simulink model "drone"  (Simulink 8.5)
settings: Solver=ode45  StartTime=0.0  StopTime=tsim  RelTol=1e-8  AbsTol=1e-12
undefined symbols (not defined in the file or in its folder): A, a_noise_seed, a_noise_var, a_scale, Cd, dx_init, enu2ecef, g, GPS_DT, GuideDt, h_noise_seed, h_noise_var, I, I_motor, IMU_DT, KaQ, KaR, KDhover, KIhover, Kir, KPhover, Kpr, Kpv, KQ, KR, KthQ, KthR, m, mag_bias, MAG_DT, mag_noise_seed, mag_noise_var, MaxPropRate, MaxPwmWidth, mean_a_bias, mean_w_bias, MinPwmWidth, mtow, P_init, Q, q0, qInit, R, r0, r1, r2, r3, r4, r_gps, RateToForce, Re, rho, Rmag, RunUpLimit, RunUpStartThrottle, tc, v0, v_noise_seed, v_noise_var, vc ... (+7)
libraries: simulink x13, SimLib x3
(part 2 of 2)

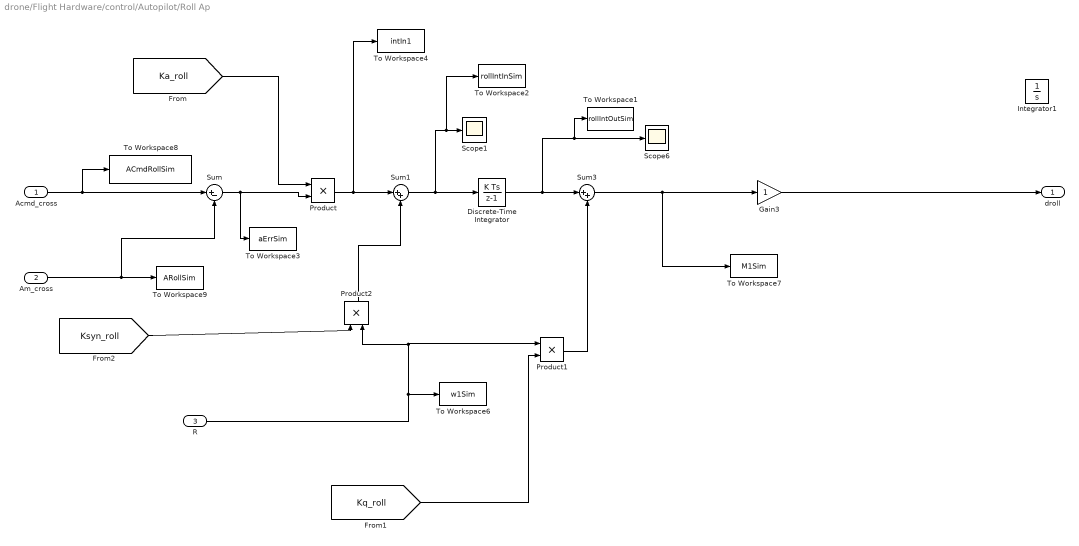
== system drone/Flight Hardware/control/Autopilot/Roll Ap ==
  Acmd_cross : Inport
  Am_cross : Inport  Port=2
  R : Inport  Port=3
  Discrete-Time Integrator : DiscreteIntegrator  InitialConditionSetting=State (most efficient)  SampleTime=IMU_DT
  Gain3 : Gain
  Integrator1 : Integrator
  Product : Product
  Product1 : Product
  Product2 : Product
  Scope1 : Scope
      settings: TimeRange=50  YMin=-10  YMax=8  SaveName=ScopeData15
  Scope6 : Scope
      settings: TimeRange=50  YMin=-0.005  YMax=0.03  SaveName=ScopeData115
  Sum : Sum  Inputs=|+-
  Sum1 : Sum  Inputs=|++
  Sum3 : Sum  Inputs=|++
  To Workspace1 : ToWorkspace  VariableName=rollIntOutSim  SampleTime=-1
  To Workspace2 : ToWorkspace  VariableName=rollIntInSim  SampleTime=-1
  To Workspace3 : ToWorkspace  VariableName=aErrSim  SampleTime=-1
  To Workspace4 : ToWorkspace  VariableName=intIn1  SampleTime=-1
  To Workspace6 : ToWorkspace  VariableName=w1Sim  SampleTime=-1
  To Workspace7 : ToWorkspace  VariableName=M1Sim  SampleTime=-1
  To Workspace8 : ToWorkspace  VariableName=ACmdRollSim  SampleTime=-1
  To Workspace9 : ToWorkspace  VariableName=ARollSim  SampleTime=-1
  droll : Outport
  wires:
  Am_cross/1 -> Sum/2, To Workspace9/1
  Product2/1 -> Sum1/2
  Sum1/1 -> Discrete-Time Integrator/1, To Workspace2/1, Scope1/1
  Product/1 -> To Workspace4/1, Sum1/1
  Discrete-Time Integrator/1 -> To Workspace1/1, Scope6/1, Sum3/1
  Product1/1 -> Sum3/2
  Sum3/1 -> To Workspace7/1, Gain3/1
  [Ka_roll] -> Product/1
  [Kq_roll] -> Product1/2
  R/1 -> To Workspace6/1, Product1/1, Product2/2
  [Ksyn_roll] -> Product2/1
  Acmd_cross/1 -> To Workspace8/1, Sum/1
  Gain3/1 -> droll/1
  Sum/1 -> To Workspace3/1, Product/2

== system drone/Flight Hardware/control/Autopilot/Throttle  ==
  ac : Inport
  am : Inport  Port=2
  Dot Product : DotProduct  InputSameDT=on  OutDataTypeStr=Inherit: Inherit via internal rule
  RunUp : Subsystem
  RunUp Logic : Subsystem
  Saturation : Saturate  UpperLimit=1  LowerLimit=0
  Scope{,1..3} (4 alike) : Scope
      Scope settings: TimeRange=10  YMin=0  YMax=0.2  SaveName=ScopeData2
      Scope1 settings: TimeRange=10  YMin=0.12445  YMax=0.13755  SaveName=ScopeData3
      Scope2 settings: TimeRange=10  YMin=9.7  YMax=11  SaveName=ScopeData68
      Scope3 settings: TimeRange=10  YMin=-106  YMax=-83  SaveName=ScopeData122
  Slope : Subsystem
  Sqrt : Sqrt  SaturateOnIntegerOverflow=on
  Step : Step  Time=15  Before=12  After=8  SampleTime=0.01
  Sum : Sum  Inputs=|++  AccumDataTypeStr=double  OutDataTypeStr=double
  To Workspace1 : ToWorkspace  VariableName=ThrottleSim  SampleTime=-1
  Throttle Cmd : Outport
  wires:
  Dot Product/1 -> Sqrt/1
  am/1 -> Dot Product/1, Dot Product/2
  RunUp Logic/2(runup x) -> Scope/1, RunUp/1(runUp)
  RunUp Logic/1(throttle x) -> Slope/3(runup)
  Sqrt/1 -> Scope2/1, RunUp Logic/1(am)
  RunUp/1(Out1) -> Scope1/1, Slope/2(RunUpValue), Sum/2
  Saturation/1 -> To Workspace1/1, Throttle Cmd/1
  Slope/1(Out1) -> Sum/1
  Sum/1 -> Scope3/1, Saturation/1
  ac/1 -> Slope/1(ac)

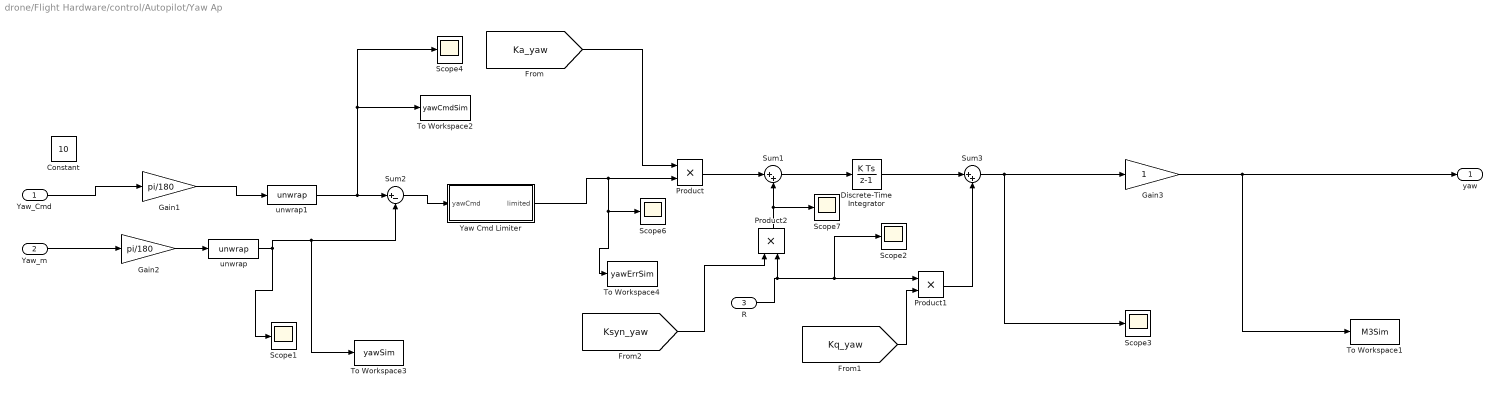
== system drone/Flight Hardware/control/Autopilot/Yaw Ap ==
  Yaw_Cmd : Inport
  Yaw_m : Inport  Port=2
  R : Inport  Port=3
  Constant : Constant  Value=10  SampleTime=IMU_DT
  Discrete-Time Integrator : DiscreteIntegrator  InitialConditionSetting=State (most efficient)  SampleTime=-1
  Gain1 : Gain  Gain=pi/180
  Gain2 : Gain  Gain=pi/180
  Gain3 : Gain
  Product : Product
  Product1 : Product
  Product2 : Product
  Scope{1..4,6..7} (6 alike) : Scope
      Scope1 settings: TimeRange=200  YMin=-0.05  YMax=0.4  SaveName=ScopeData15
      Scope2 settings: TimeRange=50  YMin=-2.5  YMax=37.5  SaveName=ScopeData48
      Scope3 settings: TimeRange=10  YMin=-7.034559643255292  YMax=12.94314381270903  SaveName=ScopeData12
      Scope4 settings: TimeRange=20  YMin=-0.006  YMax=0.006  SaveName=ScopeData119
      Scope6 settings: TimeRange=20  YMin=-0.006  YMax=0.006  SaveName=ScopeData52
      Scope7 settings: TimeRange=50  YMin=-2.5  YMax=37.5  SaveName=ScopeData53
  Sum1 : Sum  Inputs=|++
  Sum2 : Sum  Inputs=|+-
  Sum3 : Sum  Inputs=|++
  To Workspace1 : ToWorkspace  VariableName=M3Sim  SampleTime=-1
  To Workspace2 : ToWorkspace  VariableName=yawCmdSim  SampleTime=-1
  To Workspace3 : ToWorkspace  VariableName=yawSim  SampleTime=-1
  To Workspace4 : ToWorkspace  VariableName=yawErrSim  SampleTime=-1
  Yaw Cmd Limiter : Subsystem
  unwrap : SimLib/unwrap
  unwrap1 : SimLib/unwrap
  yaw : Outport
  wires:
  Product2/1 -> Scope7/1, Sum1/2
  Sum1/1 -> Discrete-Time Integrator/1
  Product/1 -> Sum1/1
  Discrete-Time Integrator/1 -> Sum3/1
  Product1/1 -> Sum3/2
  Sum3/1 -> Gain3/1, Scope3/1
  Gain3/1 -> To Workspace1/1, yaw/1
  [Ka_yaw] -> Product/1
  [Kq_yaw] -> Product1/2
  R/1 -> Product2/2, Scope2/1, Product1/1
  [Ksyn_yaw] -> Product2/1
  unwrap/1 -> To Workspace3/1, Sum2/2, Scope1/1
  unwrap1/1 -> Scope4/1, To Workspace2/1, Sum2/1
  Gain1/1 -> unwrap1/1
  Gain2/1 -> unwrap/1
  Yaw_m/1 -> Gain2/1
  Yaw_Cmd/1 -> Gain1/1
  Sum2/1 -> Yaw Cmd Limiter/1(yawCmd)
  Yaw Cmd Limiter/1("limited ") -> To Workspace4/1, Scope6/1, Product/2

== system drone/Flight Hardware/control/Guidance/v1 cmd ==
  r : Inport
  v : Inport  Port=2
  rc : Inport  Port=3
  vc : Inport  Port=4
  Embedded MATLAB Function2 : MATLAB Function  TreatAsAtomicUnit=on
  Gain : Gain  Gain=a_scale
  Mux1 : Mux  Inputs=2
  Scope{1..5,8} (6 alike) : Scope
      Scope1 settings: TimeRange=140  YMin=9.675  YMax=9.95  SaveName=ScopeData23
      Scope2 settings: TimeRange=2.391750639737455  YMin=-0.00131617173055854  YMax=0.0006389084610017104  SaveName=ScopeData117
      Scope3 settings: TimeRange=80  YMin=-0.5  YMax=10  SaveName=ScopeData31
      Scope4 settings: TimeRange=140  YMin=8  YMax=24  SaveName=ScopeData39
      Scope5 settings: TimeRange=140  YMin=-5e+09  YMax=1e+10  SaveName=ScopeData84
      Scope8 settings: TimeRange=140  YMin=8.75  YMax=9.5  SaveName=ScopeData114
  Subsystem : Subsystem
  Subsystem2 : Subsystem
  Subsystem3 : Subsystem
  Sum4 : Sum  Inputs=+++
  To Workspace1 : ToWorkspace  VariableName=vErr  SampleTime=-1
  To Workspace2 : ToWorkspace  VariableName=rErr  SampleTime=-1
  To Workspace3 : ToWorkspace  VariableName=aCurve  SampleTime=-1
  To Workspace4 : ToWorkspace  VariableName=hErr  SampleTime=-1
  To Workspace5 : ToWorkspace  VariableName=vH  SampleTime=-1
  To Workspace6 : ToWorkspace  VariableName=accelCmd  SampleTime=-1
  To Workspace7 : ToWorkspace  VariableName=hAccelCmd  SampleTime=-1
  acmd : Outport
  f tot : Outport  Port=2
  wires:
  Subsystem/1(ftot) -> Mux1/2, To Workspace7/1, Scope1/1
  Sum4/1 -> Mux1/1
  r/1 -> Subsystem3/1(r)
  rc/1 -> Subsystem3/2(rc)
  v/1 -> Subsystem3/4(v)
  vc/1 -> Subsystem3/3(vc)
  Subsystem3/4(herr) -> To Workspace4/1, Subsystem/1(herr), Scope5/1
  Subsystem3/3(acurve) -> To Workspace3/1, Sum4/3, Scope8/1
  Subsystem3/1(eR) -> To Workspace2/1, Subsystem2/1(eP)
  Embedded MATLAB Function2/1(ftot) -> f tot/1, Scope4/1
  Gain/1 -> Embedded MATLAB Function2/1(acmd), acmd/1
  Mux1/1 -> Gain/1, Scope3/1
  Subsystem3/2("ev ") -> To Workspace1/1, Subsystem2/2(v)
  Subsystem2/1(vc) -> To Workspace6/1, Sum4/1
  Subsystem3/5(vh) -> To Workspace5/1, Subsystem/2(vh)

== system drone/Flight Hardware/state estimator1/Subsystem/solve direction cosine matrix ==
  quat : Inport
  C11 : Fcn  Expr=1-(2*u[2]*u[2]) - (2*u[3]*u[3])
  C12 : Fcn  Expr=2*( u[1]*u[2] - u[3]*u[4])
  C13 : Fcn  Expr=2*( u[3]*u[1] + u[2]*u[4])
  C21 : Fcn  Expr=2*( u[1]*u[2] + u[3]*u[4])
  C22 : Fcn  Expr=1-(2*u[1]*u[1]) - (2*u[3]*u[3])
  C23 : Fcn  Expr=2*( u[3]*u[2] - u[1]*u[4])
  C31 : Fcn  Expr=2*( u[1]*u[3] - u[2]*u[4])
  C32 : Fcn  Expr=2*( u[3]*u[2] + u[1]*u[4])
  C33 : Fcn  Expr=1-(2*u[2]*u[2]) - (2*u[1]*u[1])
  Gain1 : Gain  Gain=180/pi
  Gain2 : Gain  Gain=-1
  Gain3 : Gain  Gain=-1
  MATLAB Function : MATLAB Function  TreatAsAtomicUnit=on
  Mux : Mux  Inputs=3
  nutation : Trigonometry  Operator=asin
  precession : Trigonometry  Operator=atan2
  spin : Trigonometry  Operator=atan2
  C : Outport
  roll pitch yaw : Outport  Port=2
  wires:
  quat/1 -> C13/1, C11/1, C12/1, C21/1, C22/1, C23/1, C31/1, C33/1, C32/1
  C11/1 -> MATLAB Function/1(C11)
  C12/1 -> MATLAB Function/2(C12), Gain2/1
  C13/1 -> MATLAB Function/3(C13)
  C21/1 -> MATLAB Function/4(C21)
  C22/1 -> MATLAB Function/5(C22), spin/2
  C23/1 -> MATLAB Function/6(C23)
  C31/1 -> MATLAB Function/7(C31), Gain3/1
  C32/1 -> MATLAB Function/8(C32), nutation/1
  C33/1 -> MATLAB Function/9(C33), precession/2
  Gain1/1 -> roll pitch yaw/1
  Mux/1 -> Gain1/1
  Gain2/1 -> spin/1
  Gain3/1 -> precession/1
  nutation/1 -> Mux/1
  spin/1 -> Mux/3
  precession/1 -> Mux/2
  MATLAB Function/1(R) -> C/1

== system drone/Physics Modeling/Equations of Motion/Subsystem/solve direction cosine matrix ==
  quat : Inport
  C11 : Fcn  Expr=1-(2*u[2]*u[2]) - (2*u[3]*u[3])
  C12 : Fcn  Expr=2*( u[1]*u[2] - u[3]*u[4])
  C13 : Fcn  Expr=2*( u[3]*u[1] + u[2]*u[4])
  C21 : Fcn  Expr=2*( u[1]*u[2] + u[3]*u[4])
  C22 : Fcn  Expr=1-(2*u[1]*u[1]) - (2*u[3]*u[3])
  C23 : Fcn  Expr=2*( u[3]*u[2] - u[1]*u[4])
  C31 : Fcn  Expr=2*( u[1]*u[3] - u[2]*u[4])
  C32 : Fcn  Expr=2*( u[3]*u[2] + u[1]*u[4])
  C33 : Fcn  Expr=1-(2*u[2]*u[2]) - (2*u[1]*u[1])
  Gain1 : Gain  Gain=360/(2*pi)
  Gain2 : Gain  Gain=-1
  Gain3 : Gain  Gain=-1
  MATLAB Function : MATLAB Function  TreatAsAtomicUnit=on
  Mux : Mux  Inputs=3
  nutation : Trigonometry  Operator=asin
  precession : Trigonometry  Operator=atan2
  spin : Trigonometry  Operator=atan2
  C : Outport
  roll pitch yaw : Outport  Port=2
  wires:
  quat/1 -> C13/1, C11/1, C12/1, C21/1, C22/1, C23/1, C31/1, C33/1, C32/1
  C11/1 -> MATLAB Function/1(C11)
  C12/1 -> MATLAB Function/2(C12), Gain2/1
  C13/1 -> MATLAB Function/3(C13)
  C21/1 -> MATLAB Function/4(C21)
  C22/1 -> MATLAB Function/5(C22), spin/2
  C23/1 -> MATLAB Function/6(C23)
  C31/1 -> MATLAB Function/7(C31), Gain3/1
  C32/1 -> MATLAB Function/8(C32), nutation/1
  C33/1 -> MATLAB Function/9(C33), precession/2
  Gain1/1 -> roll pitch yaw/1
  Mux/1 -> Gain1/1
  Gain2/1 -> spin/1
  Gain3/1 -> precession/1
  nutation/1 -> Mux/1
  spin/1 -> Mux/3
  precession/1 -> Mux/2
  MATLAB Function/1(R) -> C/1

== system drone/Physics Modeling/Props/Rate to Force/location moment ==
  F1 : Inport
  F2 : Inport  Port=2
  F3 : Inport  Port=3
  F4 : Inport  Port=4
  Constant : Constant  Value=r1
  Constant1 : Constant  Value=r2
  Constant2 : Constant  Value=r3
  Constant3 : Constant  Value=r4
  MATLAB Function : MATLAB Function  TreatAsAtomicUnit=on
  MATLAB Function1 : MATLAB Function  TreatAsAtomicUnit=on
  MATLAB Function2 : MATLAB Function  TreatAsAtomicUnit=on
  MATLAB Function3 : MATLAB Function  TreatAsAtomicUnit=on
  Scope{1..4} (4 alike) : Scope
      Scope1 settings: YMin=-1  YMax=1  SaveName=ScopeData17
      Scope2 settings: TimeRange=50  YMin=-1  YMax=1  SaveName=ScopeData16
      Scope3 settings: TimeRange=50  YMin=-1  YMax=1  SaveName=ScopeData18
      Scope4 settings: TimeRange=50  YMin=-1  YMax=1  SaveName=ScopeData19
  Sum : Sum  Inputs=++++
  M : Outport
  wires:
  F2/1 -> MATLAB Function1/2(u2)
  F1/1 -> MATLAB Function/2(u2)
  Constant/1 -> MATLAB Function/1(u1)
  Sum/1 -> M/1
  MATLAB Function/1(y) -> Scope2/1, Sum/1
  MATLAB Function1/1(y) -> Sum/2, Scope1/1
  MATLAB Function2/1(y) -> Scope3/1, Sum/3
  MATLAB Function3/1(y) -> Sum/4, Scope4/1
  Constant1/1 -> MATLAB Function1/1(u1)
  Constant2/1 -> MATLAB Function2/1(u1)
  F3/1 -> MATLAB Function2/2(u2)
  F4/1 -> MATLAB Function3/2(u2)
  Constant3/1 -> MATLAB Function3/1(u1)

== system drone/Physics Modeling/Props/Rate to Force/location moment1 ==
  F : Inport
  Constant : Constant  Value=0
  Mux : Mux  Inputs=3
  F1 : Outport
  wires:
  Constant/1 -> Mux/2, Mux/1
  F/1 -> Mux/3
  Mux/1 -> F1/1

== system drone/Physics Modeling/Props/Rate to Force/location moment2 ==
  F : Inport
  Constant : Constant  Value=0
  Mux : Mux  Inputs=3
  F1 : Outport
  wires:
  Constant/1 -> Mux/2, Mux/1
  F/1 -> Mux/3
  Mux/1 -> F1/1

== system drone/Physics Modeling/Props/Rate to Force/location moment3 ==
  F : Inport
  Constant : Constant  Value=0
  Mux : Mux  Inputs=3
  F1 : Outport
  wires:
  Constant/1 -> Mux/2, Mux/1
  F/1 -> Mux/3
  Mux/1 -> F1/1

== system drone/Physics Modeling/Props/Rate to Force/location moment4 ==
  F : Inport
  Constant : Constant  Value=0
  Mux : Mux  Inputs=3
  F1 : Outport
  wires:
  Constant/1 -> Mux/2, Mux/1
  F/1 -> Mux/3
  Mux/1 -> F1/1

== system drone/Physics Modeling/Props/Rate to Force2/Motor 1 ==
  w1 : Inport
  Constant : Constant  Value=0
  Gain : Gain
  Mux : Mux  Inputs=3
  M : Outport
  wires:
  Mux/1 -> M/1
  Constant/1 -> Mux/2, Mux/1
  Gain/1 -> Mux/3
  w1/1 -> Gain/1

== system drone/Physics Modeling/Props/Rate to Force2/Motor 2 ==
  w2 : Inport
  Constant : Constant  Value=0
  Gain : Gain
  Mux : Mux  Inputs=3
  M : Outport
  wires:
  Mux/1 -> M/1
  Constant/1 -> Mux/2, Mux/1
  Gain/1 -> Mux/3
  w2/1 -> Gain/1

== system drone/Physics Modeling/Props/Rate to Force2/Motor 3 ==
  w3 : Inport
  Constant : Constant  Value=0
  Gain : Gain
  Mux : Mux  Inputs=3
  M : Outport
  wires:
  Mux/1 -> M/1
  Constant/1 -> Mux/2, Mux/1
  Gain/1 -> Mux/3
  w3/1 -> Gain/1

== system drone/Physics Modeling/Props/Rate to Force2/Motor 4 ==
  w4 : Inport
  Constant : Constant  Value=0
  Gain : Gain
  Mux : Mux  Inputs=3
  M : Outport
  wires:
  Mux/1 -> M/1
  Constant/1 -> Mux/2, Mux/1
  Gain/1 -> Mux/3
  w4/1 -> Gain/1

== system drone/Flight Hardware/control/Autopilot/Calc Frames/LPF ==
  quat : Inport
  Gain1 : Gain
  Gain2 : Gain  Gain=0
  Scope1 : Scope
      settings: TimeRange=80  YMin=-0.2  YMax=1.2  SaveName=ScopeData82
  Scope2 : Scope
      settings: TimeRange=30  YMin=-40  YMax=40  SaveName=ScopeData83
  Sum : Sum  Inputs=|++
  Unit Delay : UnitDelay  InitialCondition=[0 0 0 1]  SampleTime=-1
  qout : Outport
  wires:
  Gain1/1 -> Sum/1
  Gain2/1 -> Sum/2
  quat/1 -> Scope2/1, Gain1/1
  Sum/1 -> Scope1/1, Unit Delay/1, qout/1
  Unit Delay/1 -> Gain2/1

== system drone/Flight Hardware/control/Autopilot/Calc Frames/Subsystem ==
  note: Based on Prof Howell AAE 440 Notes
  note: C is row notation so transpose it!
  quat : Inport
  Permute Dimensions : PermuteDimensions
  To Workspace2 : ToWorkspace  VariableName=Ctest  SampleTime=IMU_DT
  solve direction cosine matrix : Subsystem
  angles : Outport
  dcm_c2b : Outport  Port=2
  wires:
  quat/1 -> solve direction cosine matrix/1(quat)
  solve direction cosine matrix/2(roll pitch yaw) -> angles/1
  solve direction cosine matrix/1(C) -> Permute Dimensions/1, To Workspace2/1
  Permute Dimensions/1 -> dcm_c2b/1

== system drone/Flight Hardware/control/Autopilot/Calc Frames/YAW CMD ==
  v : Inport
  Constant : Constant  Value=-180*pi/180  SampleTime=IMU_DT
  Demux : Demux  Outputs=2
  Manual Switch : ManualSwitch
  To Workspace3 : ToWorkspace  VariableName=Vc  SampleTime=IMU_DT
  To Workspace4 : ToWorkspace  VariableName=Vc1  SampleTime=IMU_DT
  Trigonometric Function : Trigonometry  Operator=atan2
  unwrap : SimLib/unwrap
  yawcmd : Outport
  wires:
  v/1 -> Demux/1
  Demux/2 -> To Workspace4/1, Trigonometric Function/1
  Demux/1 -> To Workspace3/1, Trigonometric Function/2
  Constant/1 -> Manual Switch/2
  Manual Switch/1 -> yawcmd/1
  Trigonometric Function/1 -> unwrap/1
  unwrap/1 -> Manual Switch/1

== system drone/Flight Hardware/control/Autopilot/Throttle /RunUp ==
  runUp : Inport
  Constant : Constant  Value=0.001/IMU_DT
  Discrete-Time Integrator : DiscreteIntegrator  InitialCondition=RunUpStartThrottle  InitialConditionSetting=State (most efficient)  SampleTime=-1
  Product : Product
  Out1 : Outport
  wires:
  Constant/1 -> Product/1
  runUp/1 -> Product/2
  Discrete-Time Integrator/1 -> Out1/1
  Product/1 -> Discrete-Time Integrator/1

== system drone/Flight Hardware/control/Autopilot/Throttle /RunUp Logic ==
  am : Inport
  Compare To Constant : simulink/Logic and Bit Operations/Compare To Constant  relop=<=  const=RunUpLimit  OutDataTypeStr=uint8
  Compare To Zero : simulink/Logic and Bit Operations/Compare To Zero  relop===  OutDataTypeStr=boolean
  Logical Operator : Logic  AllPortsSameDT=off  OutDataTypeStr=boolean
  Scope : Scope
      settings: SaveName=ScopeData20
  Scope1 : Scope
      settings: YMin=80.3  YMax=80.36  SaveName=ScopeData40
  Unit Delay : UnitDelay  InitialCondition=1  SampleTime=-1
  throttle x : Outport  OutMin=[0]  OutMax=[1]  PortDimensions=1
  runup x : Outport  Port=2  PortDimensions=1
  wires:
  Compare To Constant/1 -> Logical Operator/1
  Logical Operator/1 -> Unit Delay/1, runup x/1, Compare To Zero/1
  Unit Delay/1 -> Logical Operator/2
  Compare To Zero/1 -> throttle x/1, Scope/1
  am/1 -> Scope1/1, Compare To Constant/1

== system drone/Flight Hardware/control/Autopilot/Throttle /Slope ==
  ac : Inport
  RunUpValue : Inport  Port=2
  runup : Inport  Port=3
  Constant : Constant  Value=RunUpLimit
  Gain : Gain  Gain=1/RunUpLimit
  Product : Product  Inputs=***
  Product1 : Product
  Scope2 : Scope
      settings: TimeRange=10  YMin=9.7  YMax=11  SaveName=ScopeData129
  Sum : Sum  Inputs=|+-
  Out1 : Outport
  tag scope: Throttle2Force=global
  wires:
  RunUpValue/1 -> Gain/1
  Gain/1 -> Product1/1, Product/2
  ac/1 -> Sum/1
  Constant/1 -> Sum/2
  Sum/1 -> Product/1
  runup/1 -> Product1/2, Product/3
  Product/1 -> Out1/1
  Product1/1 -> Scope2/1, [Throttle2Force]

== system drone/Flight Hardware/control/Autopilot/Yaw Ap/Yaw Cmd Limiter ==
  yawCmd : Inport
  Saturation : Saturate  UpperLimit=20*pi/180  LowerLimit=-20*pi/180
  Scope1 : Scope
      settings: YMin=-0.4  YMax=0.4  SaveName=ScopeData120
  Scope2 : Scope
      settings: YMin=-4  YMax=4  SaveName=ScopeData121
  Sum1 : Sum  Inputs=|++
  "limited " : Outport
  wires:
  Sum1/1 -> "limited "/1
  Saturation/1 -> Scope1/1, Sum1/1
  yawCmd/1 -> Scope2/1, Saturation/1

== system drone/Flight Hardware/control/Guidance/v1 cmd/Subsystem ==
  herr : Inport
  vh : Inport  Port=2
  Discrete-Time Integrator : DiscreteIntegrator  SampleTime=GuideDt
  Gain : Gain
  Gain1 : Gain  Gain=-1
  Gain2 : Gain  Gain=KPhover
  Gain3 : Gain  Gain=KIhover
  Gain4 : Gain  Gain=KDhover
  Scope{1..4} (4 alike) : Scope
      Scope1 settings: TimeRange=100  YMin=9.6  YMax=10.65  SaveName=ScopeData67
      Scope2 settings: TimeRange=100  YMin=-0.000103  YMax=-9e-005  SaveName=ScopeData22
      Scope3 settings: TimeRange=100  YMin=9.6  YMax=10.65  SaveName=ScopeData50
      Scope4 settings: TimeRange=20  YMin=0  YMax=10  SaveName=ScopeData86
  Sum : Sum  Inputs=|++  OutDataTypeStr=Inherit: Same as first input
  Sum2 : Sum  Inputs=+++
  ftot : Outport
  wires:
  Gain2/1 -> Sum2/1
  Discrete-Time Integrator/1 -> Gain3/1
  Gain3/1 -> Sum2/2, Scope1/1
  Gain4/1 -> Scope2/1, Sum2/3
  Sum2/1 -> Gain/1
  herr/1 -> Discrete-Time Integrator/1, Scope3/1, Gain2/1
  Gain/1 -> Scope4/1, Sum/1
  Sum/1 -> ftot/1
  vh/1 -> Gain1/1
  Gain1/1 -> Gain4/1

== system drone/Flight Hardware/control/Guidance/v1 cmd/Subsystem2 ==
  eP : Inport
  v : Inport  Port=2
  Discrete-Time Integrator : DiscreteIntegrator  SampleTime=GuideDt
  Gain : Gain
  Gain1 : Gain  Gain=Kpv
  Gain3 : Gain  Gain=Kpr
  Gain4 : Gain  Gain=Kir
  Scope1 : Scope
      settings: TimeRange=80  YMin=-20  YMax=12.5  SaveName=ScopeData75
  Scope3 : Scope
      settings: TimeRange=80  YMin=-6  YMax=10  SaveName=ScopeData72
  Sum1 : Sum  Inputs=+++
  vc : Outport
  wires:
  Gain/1 -> vc/1
  Sum1/1 -> Gain/1
  Gain4/1 -> Discrete-Time Integrator/1
  Gain3/1 -> Sum1/2
  Discrete-Time Integrator/1 -> Sum1/1
  eP/1 -> Gain4/1, Gain3/1, Scope3/1
  Gain1/1 -> Sum1/3
  v/1 -> Scope1/1, Gain1/1

== system drone/Flight Hardware/control/Guidance/v1 cmd/Subsystem3 ==
  r : Inport
  rc : Inport  Port=2
  vc : Inport  Port=3
  v : Inport  Port=4
  Demux1 : Demux  Outputs=3
  Demux3 : Demux  Outputs=3
  Embedded MATLAB Function1 : MATLAB Function  TreatAsAtomicUnit=on
  Mux1 : Mux  Inputs=2
  Mux3 : Mux  Inputs=2
  Scope{1..5} (5 alike) : Scope
      Scope1 settings: TimeRange=140  YMin=-0.1  YMax=0.2  SaveName=ScopeData77
      Scope2 settings: TimeRange=140  YMin=-1  YMax=10  SaveName=ScopeData81
      Scope3 settings: TimeRange=140  YMin=-1  YMax=10  SaveName=ScopeData74
      Scope4 settings: TimeRange=80  YMin=-0.75  YMax=1.25  SaveName=ScopeData65
      Scope5 settings: TimeRange=80  YMin=-2  SaveName=ScopeData66
  Sum1 : Sum  Inputs=-+
  Sum2 : Sum  Inputs=-+
  To Workspace1 : ToWorkspace  VariableName=posError  SampleTime=-1
  To Workspace7 : ToWorkspace  VariableName=VelError  SampleTime=-1
  Unit Delay : UnitDelay  SampleTime=-1
  Unit Delay1 : UnitDelay  SampleTime=-1
  eR : Outport
  "ev " : Outport  Port=2
  acurve : Outport  Port=3
  herr : Outport  Port=4
  vh : Outport  Port=5
  wires:
  Demux1/1 -> Mux3/1
  Demux1/2 -> Mux3/2
  v/1 -> Demux1/1
  vc/1 -> Embedded MATLAB Function1/1(v), Sum2/2
  rc/1 -> Sum1/2, Scope5/1, Unit Delay1/1, Embedded MATLAB Function1/2(r)
  r/1 -> Sum1/1
  Unit Delay/1 -> Embedded MATLAB Function1/4(rm2)
  Embedded MATLAB Function1/1(acurve) -> acurve/1, Scope2/1
  Embedded MATLAB Function1/2(R) -> Scope3/1
  Unit Delay1/1 -> Unit Delay/1, Embedded MATLAB Function1/3(rm)
  Demux3/1 -> Mux1/1
  Demux3/2 -> Mux1/2
  Sum1/1 -> To Workspace1/1, Demux3/1, Scope1/1
  Demux3/3 -> herr/1
  Mux1/1 -> eR/1
  Mux3/1 -> Sum2/1
  Sum2/1 -> Scope4/1, To Workspace7/1, "ev "/1
  Demux1/3 -> vh/1

== system drone/Flight Hardware/control/Autopilot/Calc Frames/Subsystem/solve direction cosine matrix ==
  quat : Inport
  C11 : Fcn  Expr=1-(2*u[2]*u[2]) - (2*u[3]*u[3])
  C12 : Fcn  Expr=2*( u[1]*u[2] - u[3]*u[4])
  C13 : Fcn  Expr=2*( u[3]*u[1] + u[2]*u[4])
  C21 : Fcn  Expr=2*( u[1]*u[2] + u[3]*u[4])
  C22 : Fcn  Expr=1-(2*u[1]*u[1]) - (2*u[3]*u[3])
  C23 : Fcn  Expr=2*( u[3]*u[2] - u[1]*u[4])
  C31 : Fcn  Expr=2*( u[1]*u[3] - u[2]*u[4])
  C32 : Fcn  Expr=2*( u[3]*u[2] + u[1]*u[4])
  C33 : Fcn  Expr=1-(2*u[2]*u[2]) - (2*u[1]*u[1])
  Gain1 : Gain  Gain=360/(2*pi)
  Gain2 : Gain  Gain=-1
  Gain3 : Gain  Gain=-1
  MATLAB Function : MATLAB Function  TreatAsAtomicUnit=on
  Mux : Mux  Inputs=3
  nutation : Trigonometry  Operator=asin
  precession : Trigonometry  Operator=atan2
  spin : Trigonometry  Operator=atan2
  C : Outport
  roll pitch yaw : Outport  Port=2
  wires:
  quat/1 -> C13/1, C11/1, C12/1, C21/1, C22/1, C23/1, C31/1, C33/1, C32/1
  C11/1 -> MATLAB Function/1(C11)
  C12/1 -> MATLAB Function/2(C12), Gain2/1
  C13/1 -> MATLAB Function/3(C13)
  C21/1 -> MATLAB Function/4(C21)
  C22/1 -> MATLAB Function/5(C22), spin/2
  C23/1 -> MATLAB Function/6(C23)
  C31/1 -> MATLAB Function/7(C31), Gain3/1
  C32/1 -> MATLAB Function/8(C32), nutation/1
  C33/1 -> MATLAB Function/9(C33), precession/2
  Gain1/1 -> roll pitch yaw/1
  Mux/1 -> Gain1/1
  Gain2/1 -> spin/1
  Gain3/1 -> precession/1
  nutation/1 -> Mux/1
  spin/1 -> Mux/3
  precession/1 -> Mux/2
  MATLAB Function/1(R) -> C/1

== matlab function Flight Hardware/control/Autopilot/Calc Frames/MATLAB Function ==
  data: C11 input double; R output double; C12 input double; C13 input double; C21 input double; C22 input double; C23 input double; C31 input double; C32 input double; C33 input double
function R = Create3x3(C11,C12,C13,C21,C22,C23,C31,C32,C33)

R = [ C11,C12,C13; C21,C22,C23 ; C31, C32 , C33];

== matlab function Physics Modeling/Drag1/Embedded MATLAB Function ==
  data: u input double; y output double
function y = fcn(u)
%#eml

y = [ cosd(u(3)), sind(u(3)) , 0;  -sind(u(3)), cosd(u(3)) 0 ; 0 , 0 , 1];

== matlab function Flight Hardware/control/Autopilot/Calc Frames/Subsystem/solve direction cosine matrix/MATLAB Function ==
  data: C11 input double; R output double; C12 input double; C13 input double; C21 input double; C22 input double; C23 input double; C31 input double; C32 input double; C33 input double
function R = Create3x3(C11,C12,C13,C21,C22,C23,C31,C32,C33)

R = [ C11,C12,C13; C21,C22,C23 ; C31, C32 , C33];

== matlab function Physics Modeling/Equations of Motion/MATLAB Function ==
  data: u1 input double; y output double; u2 input double
function y = fcn(u1,u2)
%#codegen

y = cross(u1,u2);

== matlab function Flight Hardware/state estimator1/EKF/Embedded MATLAB Function2 ==
  data: w_b output double; u input double; r output double; v output double; q output double; a_b output double
function [w_b, r,v,q, a_b]  = BreakOutState(u)
%#eml
r = u(1:3);
v = u(4:6);
a_b = u(11:13);
w_b = u(14:16);
q = u(7:10);

== matlab function Flight Hardware/Sensor Model/GPS Model/MATLAB Function ==
  data: u1 input double; y output double; u2 input double
function y = fcn(u1,u2)
%#codegen

y = cross(u1,u2);

== matlab function Flight Hardware/state estimator1/EKF/Kalman Update1 ==
  data: P_in input double; P_update output double; dx_in input double; dx_out output double; Xcor output double; debug output double; Yg input double; Ym input double; Rmag input double; Q input double; R input double; Xstar input double; w input double; a input double; Yagps input double
function [ P_update  , dx_out , Xcor, debug] = KamanUp(P_in,  dx_in  , Yg , Ym  ,Rmag, Q , R , Xstar , w , a , Yagps ) 
coder.extrinsic('.\EKF\linearizeEOM');
coder.extrinsic('.\EKF\PredictMeasurement');
coder.extrinsic('.\EKF\PredictMag');
     
new_gps = Yg(4);
new_mag = Ym(4);
y_mtilde = [0;0;0;0;0;0];
Y_predict = [0;0;0];
dt = 1/100;
dx_up  = zeros(15,1);


Y_mm = zeros(6,1);

%% Propegate

[A G ] = linearizeEOM( dx_in  , Xstar , a ,w  );
STM = eye(15) + A*dt;
dx_prop = zeros(15,1);
%dx_prop(7:9) = angErrProp;


P_prop  = STM*P_in*STM' + G*Q*G';
corrApplied = 0;
%% Handle Updates
if new_gps ==1
  % KF Equations
    Y = Yg(1:3);
    [Y_predict C] = PredictMeasurement( Xstar , w  ) ;
    S = C*P_prop*C' + R;
    K = P_prop*C'/S;
    P_update = P_prop - K * C * P_prop;
    y_tilde = Y - Y_predict ;   
    dx_up = K*y_tilde;
   
    corrApplied = 1;
elseif new_mag == 1
     Ym1 = Ym(1:3); Ym2 = Yagps(1:3);
     Ym1 = Ym1./sqrt(dot(Ym1,Ym1));
     Ym2 = Ym2./sqrt(dot(Ym2,Ym2));
     Ymag = [Ym1 ; Ym2];
     [Y_mm Cm] = predictMag( Xstar , a);
     Sm = Cm*P_prop*Cm' + Rmag;
     Km = P_prop*Cm'/Sm;
     P_update = P_prop - Km*Cm*P_prop ;
     y_mtilde= Ymag - ( Y_mm  ); 
     dx_up = Km*y_mtilde;
     corrApplied = 1;
else
     P_update = P_prop;
end


if corrApplied==1
    
    
 
    rv_cor = Xstar(1:6) +  dx_up(1:6);
     bias_cor = Xstar(11:16)+ dx_up(10:15);
     dAngs =  dx_up(7:9) ;
     quatUp = updateQuat( Xstar(7:10) , dAngs);
     
     Xcor =[  rv_cor ; quatUp ; bias_cor  ];
     dx_out = dx_prop + dx_up;     
  
else
    dx_out =dx_prop;
    P_update = P_prop;
    Xcor = Xstar;
end


debug =[Y_predict];

== matlab function Flight Hardware/state estimator1/EKF/State Propegator ==
  data: a_in input double; w_in input double; X_minus input double; Xprop output double; debug output double
function [   Xprop ,debug ] = TimeUpdate(  a_in, w_in  , X_minus) 

   
dt = 1/100;
M = 100;

dt_up = dt/M;


rk = X_minus(1:3);
vk = X_minus(4:6);
a_b = X_minus(11:13);
w_b = X_minus(14:16);
qk = X_minus(7:10);

% Apply Correction
w_corr = w_in - w_b;
w1 = w_corr(1);w2 = w_corr(2);w3 = w_corr(3);
a = a_in-a_b;

for k = 1:M
   q1 = qk(1); q2 = qk(2); q3 = qk(3); q4 = qk(4); 

  
   
   DCM_l2b = [ 1-2*q2*q2-2*q3*q3 , 2*(q1*q2 + q3*q4) , 2*(q3*q1 - q2*q4) ;... 
               2*(q1*q2 - q3*q4) , 1 - 2*q1*q1 - 2*q3*q3 , 2*(q3*q2 + q1*q4) ;...  
               2*(q1*q3 + q2*q4) , 2*(q3*q2 - q1*q4) , 1 - 2*q2*q2 - 2*q1*q1];
   OM = [0 w3 -w2 w1 ; -w3 0 w1 w2 ; w2 -w1 0 w3 ; -w1 -w2 -w3 0 ];
   ax = DCM_l2b'*a - [0;0; 9.80665]; 
  
   vk = ax*dt_up + vk; 
   rk = rk + vk*dt_up + .5*dt_up*dt_up*ax;  
   qdot = .5*OM*qk;
   qk = qdot*dt_up + qk ;
   qk =qk./sqrt(dot(qk,qk));
   
  
   
end
   
 Xprop = [ rk ; vk ; qk ; a_b ; w_b ];

debug = 0;

== matlab function Flight Hardware/state estimator1/Subsystem/solve direction cosine matrix/MATLAB Function ==
  data: C11 input double; R output double; C12 input double; C13 input double; C21 input double; C22 input double; C23 input double; C31 input double; C32 input double; C33 input double
function R = Create3x3(C11,C12,C13,C21,C22,C23,C31,C32,C33)

R = [ C11,C12,C13; C21,C22,C23 ; C31, C32 , C33];

== matlab function Flight Hardware/Sensor Model/Mag Model1/Embedded MATLAB Function ==
  data: Mhat output double
function Mhat  = Calc_Mag_Field
%#eml


colat = 90-32.2;
Bn = -sind(colat);
Bu = -2*cosd(colat);
M = [0 Bn Bu]';

Mhat = M./sqrt(dot(M,M));
Mhat = [0 24.4 -40.6]';

== matlab function Physics Modeling/Equations of Motion/Subsystem/solve direction cosine matrix/MATLAB Function ==
  data: C11 input double; R output double; C12 input double; C13 input double; C21 input double; C22 input double; C23 input double; C31 input double; C32 input double; C33 input double
function R = Create3x3(C11,C12,C13,C21,C22,C23,C31,C32,C33)

R = [ C11,C12,C13; C21,C22,C23 ; C31, C32 , C33];

== matlab function Flight Hardware/control/Guidance/v1 cmd/Embedded MATLAB Function2 ==
  data: acmd input double; ftot output double
function ftot  = fcn( acmd)

%ftot = sqrt( dot( acmd , acmd) ) ;
ftot = acmd(3);

== matlab function Flight Hardware/control/Guidance/v1 cmd/Subsystem3/Embedded MATLAB Function1 ==
  data: v input double; r input double; rm input double; rm2 input double; acurve output double; R output double
function [acurve,R]  = fcn( v ,  r , rm , rm2  )


V = sqrt(dot(v,v));


x3 = r(1);
y3 = r(2);
x2 = rm(1);
y2 = rm(2);
x1 = rm2(1);
y1 = rm2(2);

ma = (y2-y1)/(x2-x1);
mb = (y3-y2)/(x3-x2);

x = ( ma*mb*(y1-y3) + mb*(x1+x2) - ma*(x2+x3))/(2 * ( mb-ma));
y = ( (x1+x2)/2 - x )/ma + (y1+y2)/2;

vec = [x-x3 , y-y3];
R = sqrt(dot(vec,vec)) ;
if( R > 0 && R~=inf ) 
    A = V*V./R;
    acurve = A.*( vec'./R ) ;
else
    acurve = [0  0]';
    R= 0;
end

== matlab function Physics Modeling/Props/Rate to Force/location moment/MATLAB Function ==
  data: u1 input double; y output double; u2 input double
function y = fcn(u1,u2)
%#codegen

y = cross(u1,u2);

== matlab function Physics Modeling/Props/Rate to Force/location moment/MATLAB Function1 ==
  data: u1 input double; y output double; u2 input double
function y = fcn(u1,u2)
%#codegen

y = cross(u1,u2);

== matlab function Physics Modeling/Props/Rate to Force/location moment/MATLAB Function2 ==
  data: u1 input double; y output double; u2 input double
function y = fcn(u1,u2)
%#codegen

y = cross(u1,u2);

== matlab function Physics Modeling/Props/Rate to Force/location moment/MATLAB Function3 ==
  data: u1 input double; y output double; u2 input double
function y = fcn(u1,u2)
%#codegen

y = cross(u1,u2);
